simulink library "Plane_Movement_walk_backward"  (R2024a)
settings: Solver=VariableStepAuto  StartTime=0.0  StopTime=10.0  RelTol=1e-3
undefined symbols (not defined in the file): Lower_limbs, Upper_limbs
libraries: functionAngles x1, functionBezier_backward x1
settings Model: Creator=renre  LastModifiedBy=renre

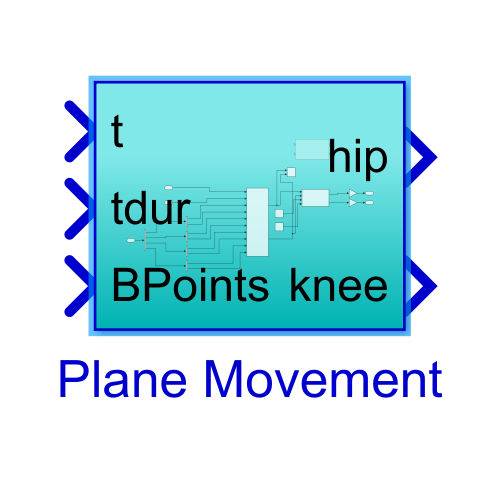
[thumbnail: Simulink's stored preview of the top-level diagram]
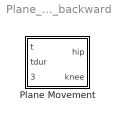
== system Plane_Movement_walk_backward ==
  Plane Movement : Subsystem

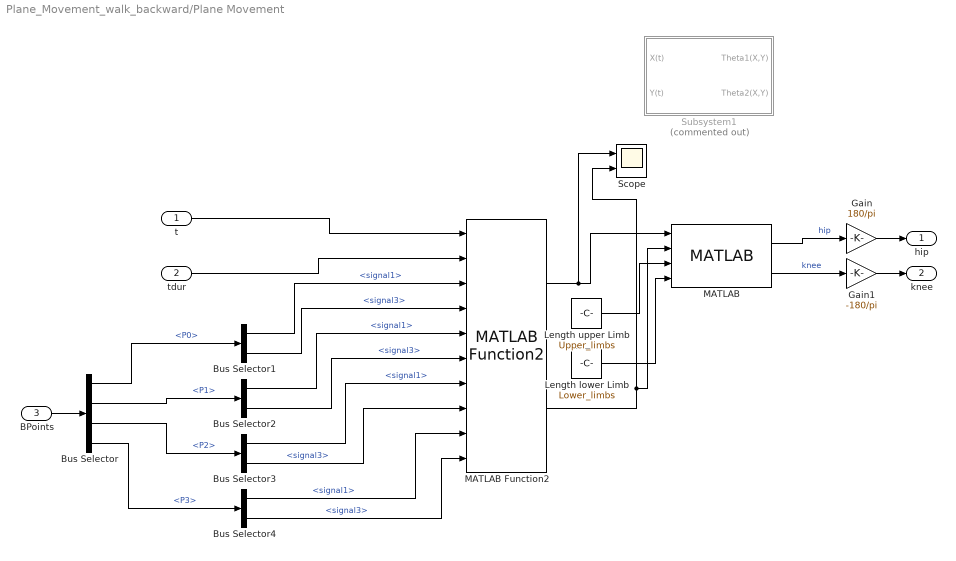
== system Plane_Movement_walk_backward/Plane Movement ==
  t : Inport
  tdur : Inport  Port=2
  BPoints : Inport  Port=3
  Bus Selector : BusSelector  OutputSignals=P0,P1,P2,P3
  Bus Selector{1..4} (4 alike) : BusSelector  OutputSignals=signal1,signal3
  Gain : Gain  Gain=180/pi
  Gain1 : Gain  Gain=-180/pi
  Length lower Limb : Constant  Value=Lower_limbs
  Length upper Limb : Constant  Value=Upper_limbs
  MATLAB : functionAngles/MATLAB  SystemSampleTime=-1  VariantActivationTime=update diagram  AllowFlexibleInterface=on  Latency=0  AutoFrameSizeCalculation=off
  MATLAB Function2 : functionBezier_backward/MATLAB Function2  SystemSampleTime=-1  VariantActivationTime=update diagram  AllowFlexibleInterface=on  Latency=0  AutoFrameSizeCalculation=off
  Scope : Scope  NumInputPorts=2
  Subsystem1 : Subsystem  Commented=on
  hip : Outport
  knee : Outport  Port=2
  wires:
  Bus Selector4/2 -> MATLAB Function2/10  "<signal3>"
  Bus Selector4/1 -> MATLAB Function2/9  "<signal1>"
  Bus Selector3/2 -> MATLAB Function2/8  "<signal3>"
  Bus Selector3/1 -> MATLAB Function2/7  "<signal1>"
  Bus Selector2/2 -> MATLAB Function2/6  "<signal3>"
  Bus Selector2/1 -> MATLAB Function2/5  "<signal1>"
  Bus Selector/4 -> Bus Selector4/1  "<P3>"
  Bus Selector/3 -> Bus Selector3/1  "<P2>"
  Bus Selector/2 -> Bus Selector2/1  "<P1>"
  Bus Selector1/2 -> MATLAB Function2/4  "<signal3>"
  Bus Selector1/1 -> MATLAB Function2/3  "<signal1>"
  Bus Selector/1 -> Bus Selector1/1  "<P0>"
  BPoints/1 -> Bus Selector/1
  Gain/1 -> hip/1
  Gain1/1 -> knee/1
  Length lower Limb/1 -> MATLAB/4
  Length upper Limb/1 -> MATLAB/3
  t/1 -> MATLAB Function2/1
  MATLAB/1 -> Gain/1  "hip"
  tdur/1 -> MATLAB Function2/2
  MATLAB/2 -> Gain1/1  "knee"
  MATLAB Function2/1 -> Scope/1, MATLAB/1
  MATLAB Function2/2 -> Scope/2, MATLAB/2

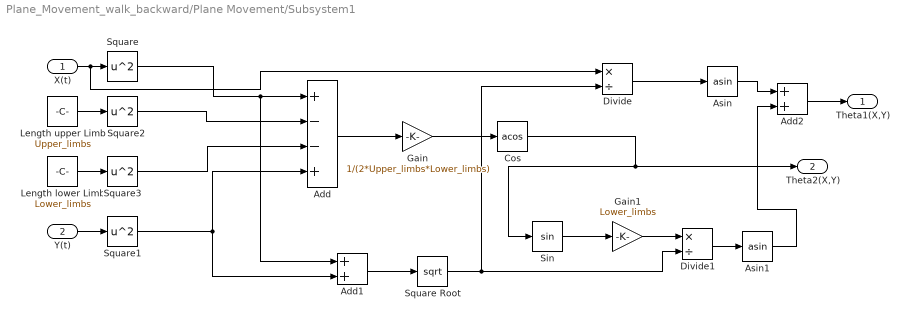
== system Plane_Movement_walk_backward/Plane Movement/Subsystem1 ==
  X(t) : Inport
  Y(t) : Inport  Port=2
  Add : Sum  Inputs=+--+
  Add1 : Sum
  Add2 : Sum
  Asin : Trigonometry  Operator=asin
  Asin1 : Trigonometry  Operator=asin
  Cos : Trigonometry  Operator=acos
  Divide : Product  Inputs=*/
  Divide1 : Product  Inputs=*/
  Gain : Gain  Gain=1/(2*Upper_limbs*Lower_limbs)
  Gain1 : Gain  Gain=Lower_limbs
  Length lower Limb : Constant  Value=Lower_limbs
  Length upper Limb : Constant  Value=Upper_limbs
  Sin : Trigonometry
  Square{,1..3} (4 alike) : Math  Operator=square
  Square Root : Sqrt
  Theta1(X,Y) : Outport
  Theta2(X,Y) : Outport  Port=2
  wires:
  Divide/1 -> Asin/1
  Add2/1 -> Theta1(X,Y)/1
  Asin1/1 -> Add2/2
  Divide1/1 -> Asin1/1
  Square Root/1 -> Divide1/2, Divide/2
  Gain1/1 -> Divide1/1
  Add1/1 -> Square Root/1
  Sin/1 -> Gain1/1
  Asin/1 -> Add2/1
  Cos/1 -> Sin/1, Theta2(X,Y)/1
  Gain/1 -> Cos/1
  Add/1 -> Gain/1
  Square1/1 -> Add/4, Add1/2
  Square3/1 -> Add/3
  Square2/1 -> Add/2
  Length lower Limb/1 -> Square3/1
  Length upper Limb/1 -> Square2/1
  Square/1 -> Add/1, Add1/1
  Y(t)/1 -> Square1/1
  X(t)/1 -> Square/1, Divide/1
